simulink model "PositionSensor"  (R2023b)
settings: Solver=VariableStepAuto  StartTime=0.0  StopTime=10.0  RelTol=1e-3
settings Model: Creator=MOHAMED  LastModifiedBy=MOHAMED
settings DataIOCC: LoadExternalInput=on

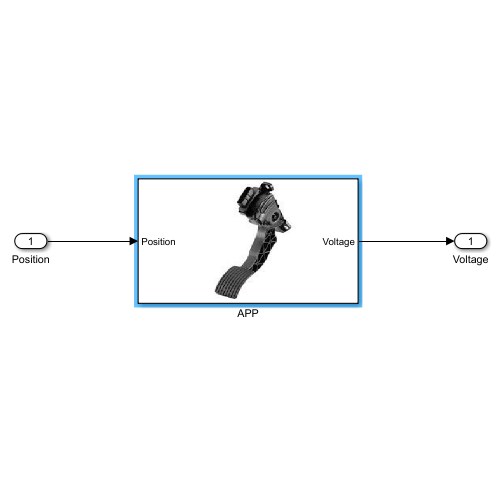
[thumbnail: Simulink's stored preview of the top-level diagram]
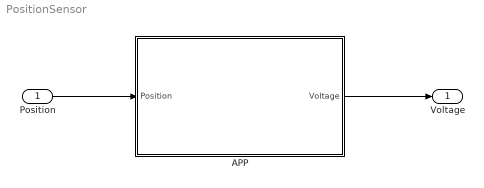
== system PositionSensor ==
  Position : Inport
  APP : Subsystem
      mask Display: image('00_Acceleration Padel Image.jpeg');
  Voltage : Outport
  wires:
  APP/1(Voltage) -> Voltage/1
  Position/1 -> APP/1(Position)

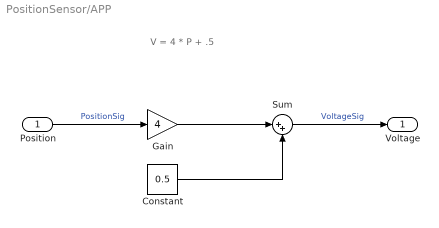
== system PositionSensor/APP ==
  note: V = 4 * P + .5
  Position : Inport
  Constant : Constant  Value=0.5
  Gain : Gain  Gain=4
  Sum : Sum  Inputs=|++
  Voltage : Outport
  wires:
  Position/1 -> Gain/1  "PositionSig"
  Gain/1 -> Sum/1
  Constant/1 -> Sum/2
  Sum/1 -> Voltage/1  "VoltageSig"
